simulink model "bp1_model2"  (R2019b)
settings: Solver=ode15s  StartTime=0.0  StopTime=2  FixedStep=0.001  RelTol=1e-9  EnableMultiTasking=on
PreLoadFcn:
  | alpha=[0.93,0.99,0.92]; x0=[0.2; -0.1; 0.1];
  | a=10.725; b=10.593; c=0.268; m0=-1.1726; m1=-0.7872;
  | ww=[1e-4 1e3]; N=13;
undefined symbols (not defined in the file or in its folder): G
libraries: cstblocks x1
settings Model: Creator=toshiba  LastModifiedBy=xuedi
settings DataIOCC: MaxDataPoints=10000  SaveFormat=Array  SignalLoggingSaveFormat=ModelDataLogs  ReturnWorkspaceOutputs=off
settings OptimizationCC: ExpressionDepthLimit=2147483647  LifeSpan=inf
settings DebuggingCC: UnderspecifiedInitializationDetection=Classic  MergeDetectMultiDrivingBlocksExec=none  FcnCallInpInsideContextMsg=warning  StateNameClashWarn=warning  SFUnexpectedBacktrackingDiag=warning  SFNoUnconditionalDefaultTransitionDiag=warning  SFExecutionAtInitializationDiag=none  ArithmeticOperatorsInVariantConditions=warning
settings HardwareCC: ProdBitPerPointer=32  ProdBitPerSizeT=32  ProdBitPerPtrDiffT=32  ProdLargestAtomicFloat=None  ProdIntDivRoundTo=Undefined  ProdEndianess=Unspecified  ProdWordSize=32  ProdHWDeviceType=32-bit Generic
settings ModelReferenceCC: PropagateSignalLabelsOutOfModel=off
settings SFSimCC: SimUseLocalCustomCode=off  CustomCodeUndefinedFunction=UseInterfaceOnly
settings RTWCC: RTWUseLocalCustomCode=off
settings CodeAppCC: StateflowObjectComments=on
settings GRTTargetCC: TargetLangStandard=C89/C90 (ANSI)  CombineOutputUpdateFcns=off  GRTInterface=on
settings ConfigComp: CovMetricSettings=dw  CovSaveCumulativeToWorkspaceVar=on  CovSaveSingleToWorkspaceVar=on  CovExternalEMLEnable=off

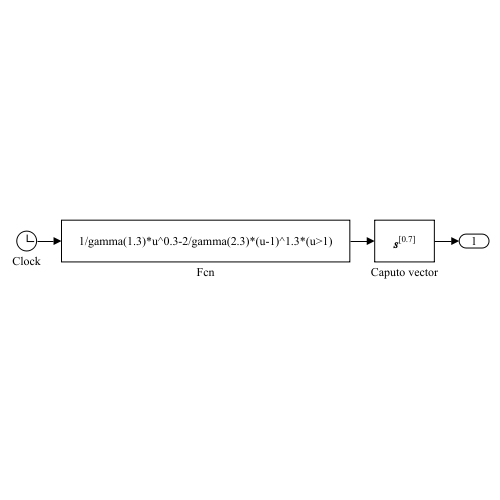
[thumbnail: Simulink's stored preview of the top-level diagram]
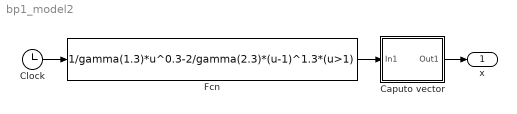
== system bp1_model2 ==
  Caputo vector : Subsystem  mask{gam=0.7, ww=ww, N=N, M=1, x0=1}
      mask prompts: gam "Derivative order gamma"; ww "Frequency range [wb,wh]"; N "Approximation order N"; M "Dimension M"; x0 "Initial condition x0"
      mask init:
      | wb=ww(1); wh=ww(2); stri=[];
      | if length(gam)==1, gam=gam*ones(M,1); end
      | for i=1:M
      |     G(i,1)=ousta_fod(1-gam(i),N,wb,wh); stri=[stri,num2str(gam(i)),','];
      | end
      | str=['{\bf{\its}}^{[' stri(1:end-1) ']}'];
      | svec2sl(gam);
      mask Display: disp(str,'texmode','on')
  Clock : Clock
  Fcn : Fcn  Expr=1/gamma(1.3)*u^0.3-2/gamma(2.3)*(u-1)^1.3*(u>1)
  x : Outport
  wires:
  Clock/1 -> Fcn/1
  Fcn/1 -> Caputo vector/1(In1)
  Caputo vector/1(Out1) -> x/1

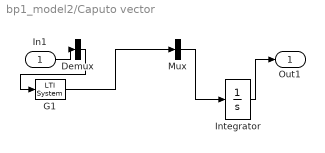
== system bp1_model2/Caputo vector ==
  In1 : Inport
  Demux : Demux  Outputs=1
  G1 : cstblocks/LTI System  sys=G(1)  IC=[]
  Integrator : Integrator  InitialCondition=x0
  Mux : Mux  Inputs=1
  Out1 : Outport
  wires:
  Demux/1 -> G1/1
  G1/1 -> Mux/1
  Integrator/1 -> Out1/1
  Mux/1 -> Integrator/1
  In1/1 -> Demux/1
